simulink model "init_subsystem_if"  (Simulink 7.0)
settings: Solver=FixedStepDiscrete  StartTime=0  StopTime=10.0  FixedStep=0.1  MaxStep=0.2  RelTol=1e-3
undefined symbols (not defined in the file or in its folder): DiscIntNeverNeededParam
settings Model: Creator=ymiyazak  LastModifiedBy=ymiyazak

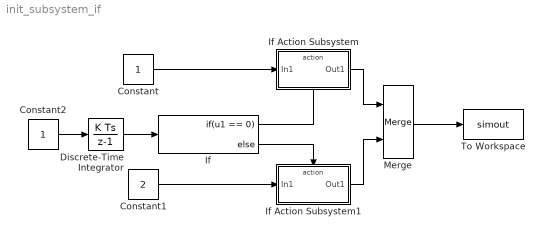
== system init_subsystem_if ==
  Constant : Constant  OutDataType=sfix(16)  OutScaling=2^0
  Constant1 : Constant  Value=2  OutDataType=sfix(16)  OutScaling=2^0
  Constant2 : Constant  OutDataType=sfix(16)  OutScaling=2^0
  Discrete-Time Integrator : DiscreteIntegrator  SampleTime=-1  OutDataType=sfix(16)  OutScaling=2^0  ICPrevOutput=DiscIntNeverNeededParam  ICPrevScaledInput=DiscIntNeverNeededParam
  If : If  IfExpression=u1 == 0
  If Action Subsystem : Subsystem  TreatAsAtomicUnit=on
  If Action Subsystem1 : Subsystem  TreatAsAtomicUnit=on
  Merge : Merge
  To Workspace : ToWorkspace  VariableName=simout  SampleTime=-1  SaveFormat=Array
  wires:
  Discrete-Time Integrator/1 -> If/1
  Constant/1 -> If Action Subsystem/1(In1)
  Constant1/1 -> If Action Subsystem1/1(In1)
  If/1 -> If Action Subsystem/Action
  If/2 -> If Action Subsystem1/Action
  If Action Subsystem/1(Out1) -> Merge/1
  If Action Subsystem1/1(Out1) -> Merge/2
  Merge/1 -> To Workspace/1
  Constant2/1 -> Discrete-Time Integrator/1

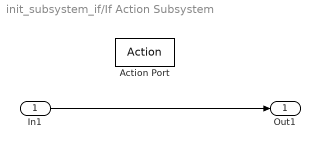
== system init_subsystem_if/If Action Subsystem ==
  In1 : Inport  OutDataType=sfix(16)  OutScaling=2^0
  Action Port : ActionPort  ActionType=then
  Out1 : Outport  OutDataType=sfix(16)  OutScaling=2^0
  wires:
  In1/1 -> Out1/1

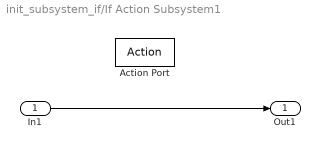
== system init_subsystem_if/If Action Subsystem1 ==
  In1 : Inport  OutDataType=sfix(16)  OutScaling=2^0
  Action Port : ActionPort  ActionType=else
  Out1 : Outport  OutDataType=sfix(16)  OutScaling=2^0
  wires:
  In1/1 -> Out1/1
